simulink model "seb_ut"  (Simulink 8.1)
settings: Solver=FixedStepDiscrete  StartTime=0.0  StopTime=10.0  FixedStep=5e-3  RelTol=1e-3
undefined symbols (not defined in the file or in its folder): KAEB_AEBAutoBrakeDecelReq_mps2
libraries: siltestlib x20, seb x1
settings Model: Creator=xsellart  LastModifiedBy=AT015411
settings DataIOCC: SignalLoggingSaveFormat=Dataset
settings OptimizationCC: ExpressionDepthLimit=128
settings DebuggingCC: FcnCallInpInsideContextMsg=EnableAllAsError
settings GRTTargetCC: CombineOutputUpdateFcns=on  GRTInterface=off

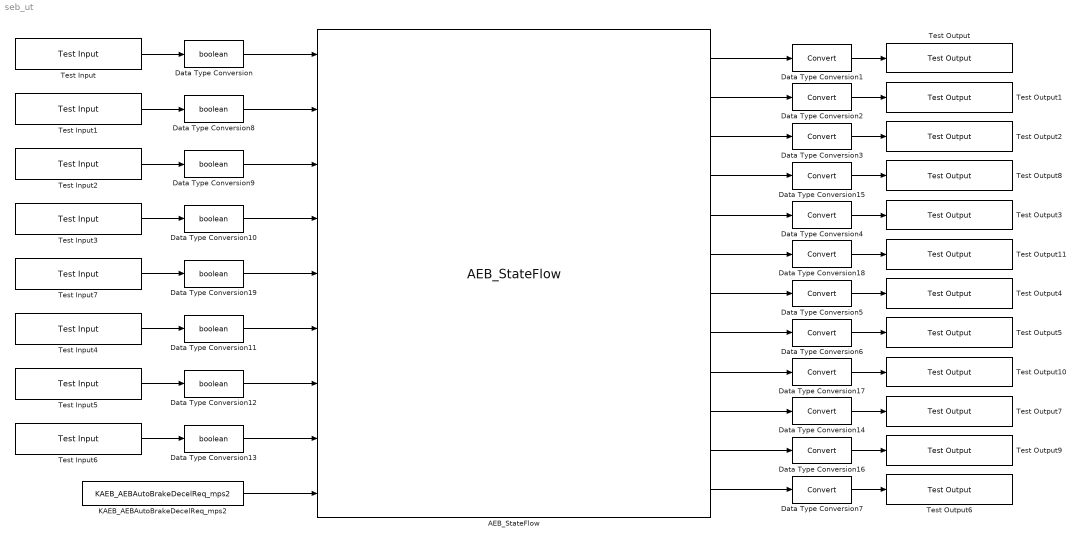
== system seb_ut ==
  AEB_StateFlow : seb/AEB_StateFlow
  Data Type Conversion{,8..13,19} (8 alike) : DataTypeConversion  OutDataTypeStr=boolean
  Data Type Conversion{1..7,14..18} (12 alike) : DataTypeConversion
  KAEB_AEBAutoBrakeDecelReq_mps2 : Constant  Value=KAEB_AEBAutoBrakeDecelReq_mps2
  Test Input : siltestlib/Test Input  varname=VJUD_AEBEnableReq_flg  sampletime=-1
  Test Input1 : siltestlib/Test Input  varname=VJUD_AEBSpeedInRange_flg  sampletime=-1
  Test Input2 : siltestlib/Test Input  varname=VJUD_AEBOperational_flg  sampletime=-1
  Test Input3 : siltestlib/Test Input  varname=VJUD_AEBActionReq_flg  sampletime=-1
  Test Input4 : siltestlib/Test Input  varname=VJUD_AEBAutoBraking_flg  sampletime=-1
  Test Input5 : siltestlib/Test Input  varname=VJUD_AEBDeactivationReq_flg  sampletime=-1
  Test Input6 : siltestlib/Test Input  varname=VIFO_BrakePedalPressed_flg  sampletime=-1
  Test Input7 : siltestlib/Test Input  varname=VJUD_AEBReturnOperational_flg  sampletime=-1
  Test Output : siltestlib/Test Output  varname=VAEB_AEBSystemState_enum  sampletime=-1
  Test Output1 : siltestlib/Test Output  varname=VAEB_AEBStateHMI_enum  sampletime=-1
  Test Output10 : siltestlib/Test Output  varname=VAEB_AEBDecelReqAppl_flg  sampletime=-1
  Test Output11 : siltestlib/Test Output  varname=VAEB_TorqueRelReqAppl_flg  sampletime=-1
  Test Output2 : siltestlib/Test Output  varname=VAEB_AEBBrakePreFillReq_flg  sampletime=-1
  Test Output3 : siltestlib/Test Output  varname=VAEB_TorqueReleaseReq_flg  sampletime=-1
  Test Output4 : siltestlib/Test Output  varname=VAEB_AEBWarningReq_flg  sampletime=-1
  Test Output5 : siltestlib/Test Output  varname=VAEB_AEBActing_flg  sampletime=-1
  Test Output6 : siltestlib/Test Output  varname=VAEB_AEBDecelReq_mps2  sampletime=-1
  Test Output7 : siltestlib/Test Output  varname=VAEB_AEBReq_flg  sampletime=-1
  Test Output8 : siltestlib/Test Output  varname=VAEB_AEBBrakePreFillReqAppl_flg  sampletime=-1
  Test Output9 : siltestlib/Test Output  varname=VAEB_AEBReqAppl_flg  sampletime=-1
  wires:
  AEB_StateFlow/1 -> Data Type Conversion1/1
  Data Type Conversion1/1 -> Test Output/1
  AEB_StateFlow/2 -> Data Type Conversion2/1
  Data Type Conversion2/1 -> Test Output1/1
  AEB_StateFlow/3 -> Data Type Conversion3/1
  Data Type Conversion3/1 -> Test Output2/1
  AEB_StateFlow/4 -> Data Type Conversion15/1
  Data Type Conversion4/1 -> Test Output3/1
  AEB_StateFlow/5 -> Data Type Conversion4/1
  Data Type Conversion5/1 -> Test Output4/1
  Data Type Conversion6/1 -> Test Output5/1
  Data Type Conversion7/1 -> Test Output6/1
  Test Input/1 -> Data Type Conversion/1
  Data Type Conversion/1 -> AEB_StateFlow/1
  Test Input1/1 -> Data Type Conversion8/1
  Data Type Conversion8/1 -> AEB_StateFlow/2
  Test Input2/1 -> Data Type Conversion9/1
  Data Type Conversion9/1 -> AEB_StateFlow/3
  Test Input3/1 -> Data Type Conversion10/1
  Data Type Conversion10/1 -> AEB_StateFlow/4
  Test Input4/1 -> Data Type Conversion11/1
  Data Type Conversion11/1 -> AEB_StateFlow/6
  Test Input5/1 -> Data Type Conversion12/1
  Data Type Conversion12/1 -> AEB_StateFlow/7
  Test Input6/1 -> Data Type Conversion13/1
  Data Type Conversion13/1 -> AEB_StateFlow/8
  Data Type Conversion14/1 -> Test Output7/1
  AEB_StateFlow/7 -> Data Type Conversion5/1
  AEB_StateFlow/9 -> Data Type Conversion17/1
  Data Type Conversion16/1 -> Test Output9/1
  AEB_StateFlow/10 -> Data Type Conversion14/1
  Data Type Conversion17/1 -> Test Output10/1
  AEB_StateFlow/8 -> Data Type Conversion6/1
  Data Type Conversion15/1 -> Test Output8/1
  AEB_StateFlow/11 -> Data Type Conversion16/1
  AEB_StateFlow/12 -> Data Type Conversion7/1
  Data Type Conversion18/1 -> Test Output11/1
  AEB_StateFlow/6 -> Data Type Conversion18/1
  Test Input7/1 -> Data Type Conversion19/1
  Data Type Conversion19/1 -> AEB_StateFlow/5
  KAEB_AEBAutoBrakeDecelReq_mps2/1 -> AEB_StateFlow/9
